simulink model "schieferFlipper"  (R2014b)
settings: Solver=ode45  StartTime=0.0  StopTime=500  RelTol=1e-3
libraries: vrlib x2
settings Model: Creator=Florian  LastModifiedBy=Florian

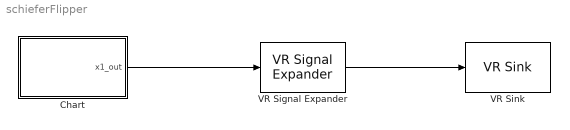
== system schieferFlipper ==
  Chart : Stateflow chart  TreatAsAtomicUnit=on
  VR Signal Expander : vrlib/VR Signal Expander  outwidth=3  outidx=[1 2]
  VR Sink : vrlib/VR Sink  InstantiateOnLoad=on  SampleTime=0.05  ViewEnable=on  RemoteChange=off  RemoteView=off  FieldsWritten=Ball.translation.3.1.1.double  WorldFileName=gegeben\Table.wrl  AutoView=off  VideoDimensions=[]  AllowVariableSize=off
  wires:
  VR Signal Expander/1 -> VR Sink/1
  Chart/1(x1_out) -> VR Signal Expander/1

== stateflow chart schieferFlipper/Chart ==
  settings: updateMethod=CONTINUOUS
  state Flipper
    during:
    %Ableitungen
    v1_dot = Acc();
    x1_dot = v1;
    %Output
    x1_out = x1;
  (default) -> Flipper : {Init}
  Flipper -> Flipper [order 1] : [Wand1Kontakt]
      | {Wand1Refl()}
  Flipper -> Flipper [order 2] : [Wand2Kontakt]
      | {Wand2Refl()}
  Flipper -> Flipper [order 3] : [Wand3Kontakt]
      | {Wand3Refl()}
  Flipper -> Flipper [order 4] : [HndKontakt]
      | {HndRefl()}
  data: a function_output; w1 function_output; w2 function_output; w3 function_output; h function_output; R constant double =0.25; RHnd constant double =0.8; v1 local double size=2,1; x1 local double size=2,1; Hnd local double size=2,1; n1 local double size=2,1; n2 local double size=2,1; n3 local double size=2,1; p1 local double size=2,1; p2 local double size=2,1; p3 local double size=2,1; p4 local double size=2,1; t1 local double size=2,1; t2 local double size=2,1; t3 local double size=2,1; x1_out output double size=2,1; g constant double =1
  data v1 settings: updateMethod=SF_CONTINUOUS_TIME_DATA
  data x1 settings: updateMethod=SF_CONTINUOUS_TIME_DATA
  function Init:
    | function Init
    | 
    | %Wand
    | p1=[0;5];
    | p2=[5;0];
    | p3=[9;0];
    | p4=[10;7];
    | 
    | %Hindernis
    | Hnd=[6;2.5];
    | 
    | %Tangentialverktoren
    | t1=(p2-p1)/norm(p2-p1);
    | t2=(p3-p2)/norm(p3-p2);
    | t3=(p4-p3)/norm(p4-p3);
    | 
    | %Normalverktoren
    | n1 = [-t1(2); t1(1)];
    | n2 = [-t2(2); t2(1)];
    | n3 = [-t3(2); t3(1)];
    | 
    | %Kugel
    | x1=[4;5];
    | v1=[0;0];
  function a=Acc:
    | function a=Acc
    |  
    | a = [0;-g]; %Beschleunigung nur in negativer Y-Richtung (Graviation)
  function w1=Wand1Kontakt:
    | function w1=Wand1Kontakt
    |  
    | richtung = v1' * n1;
    | abstand  = (x1 - p1)' * n1; %MO3b_2_post Seite 2
    |     
    | if ((abstand <= R) && (richtung < 0))
    |     w1 = true;
    | else
    |     w1 = false;
    | end
  function Wand1Refl:
    | function Wand1Refl
    |  
    | vt = v1' * t1; %Tangentialkomponente
    | vn = v1' * n1; %Normalkomponente
    | 
    | v1 = (vt' * t1) - (vn' * n1); %MOV03b 36
  function w2 = Wand2Kontakt:
    | function w2 = Wand2Kontakt
    |  
    | richtung = v1' * n2;
    | abstand = (x1 - p2)' * n2; %MO3b_2_post Seite 2
    |     
    | if ((abstand <= R) && (richtung < 0))
    |     w2 = true;
    | else
    |     w2 = false;
    | end
  function Wand2Refl:
    | function Wand2Refl
    |  
    | vt = t2' * v1; %Tangentialkomponente
    | vn = n2' * v1; %Normalkomponente
    | 
    | v1 = (vt' * t2) - (vn' * n2); %MOV03b 36
  function w3 = Wand3Kontakt:
    | function w3 = Wand3Kontakt
    |  
    | richtung = v1' * n3;
    | abstand = (x1 - p3)' * n3; %MO3b_2_post Seite 2
    |     
    | if ((abstand <= R) && (richtung < 0))
    |     w3 = true;
    | else
    |     w3 = false;
    | end
  function Wand3Refl:
    | function Wand3Refl
    |  
    | vt = t3' * v1; %Tangentialkomponente
    | vn = n3' * v1; %Normalkomponente
    | 
    | v1 = (vt' * t3) - (vn' * n3); %MOV03b 36
  function h = HndKontakt:
    | function h = HndKontakt
    |  
    | n = (x1-Hnd)/norm(x1-Hnd); %Normalvektor
    | 
    | Richtung = v1' * n;
    | 
    | if(norm(x1-Hnd)<=(R+RHnd) && Richtung<0) %MO3b_2_post Seite 4
    |     h = true;
    | else
    |     h = false;
    | end;
  function HndRefl:
    | function HndRefl
    | 
    | nHnd = (x1 - Hnd) / norm(x1 - Hnd);
    | tHnd = [nHnd(2); -nHnd(1)];
    |     
    | vt = tHnd' * v1; %Tangentialkomponente
    | vn = nHnd' * v1; %Normalkomponente
    |     
    | v1 = (vt' * tHnd) - (vn' * nHnd); %MOV03b 36
